simulink model "steady state dc motor model using speed torque relationship"  (R2021a)
settings: Solver=VariableStepAuto  StartTime=0.0  StopTime=10.0  RelTol=1e-3
settings Model: Creator=hritw  LastModifiedBy=hritw

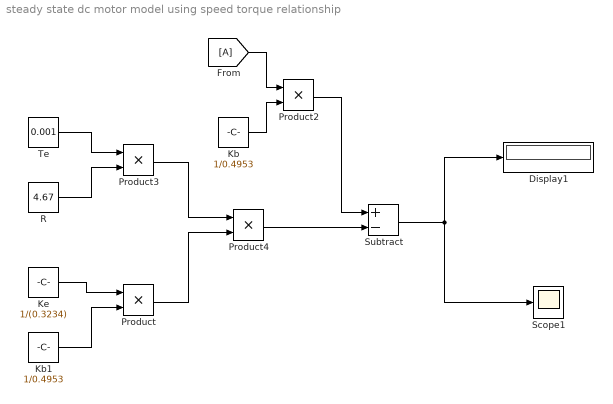
== system steady state dc motor model using speed torque relationship ==
  Display1 : Display
  Kb : Constant  Value=1/0.4953
  Kb1 : Constant  Value=1/0.4953
  Ke : Constant  Value=1/(0.3234)
  Product{,2..4} (4 alike) : Product
  R : Constant  Value=4.67
  Scope1 : Scope
  Subtract : Sum  Inputs=+-
  Te : Constant  Value=0.001
  wires:
  Kb/1 -> Product2/2
  Product2/1 -> Subtract/1
  Subtract/1 -> Display1/1, Scope1/1
  Te/1 -> Product3/1
  Product3/1 -> Product4/1
  R/1 -> Product3/2
  Ke/1 -> Product/1
  Kb1/1 -> Product/2
  Product/1 -> Product4/2
  Product4/1 -> Subtract/2
  [A] -> Product2/1
